simulink model "quad_control_outer_trainingR2015a"  (Simulink 8.5)
settings: Solver=ode45  StartTime=0.0  StopTime=40  FixedStep=0.01  MaxStep=0.1  RelTol=1e-3
InitFcn:
  | % load parameters of the default quadrotor
  | disp('Quadrotor parameters loaded by InitFcn')
  | mdl_quadrotor
  | 
  | % --- Outer loop gains --------
  | %P_X = 3.25;
  | %I_X = 0.45;
  | %D_X = 2;
  | 
  | %P_Y = 2.75;
  | %I_Y = 0.35;
  | %D_Y = 4.75;
  | 
  | %P_Z = 45;
  | %I_Z = 3.5;
  | %D_Z = 25;
  | % --------------------------
  | 
  | rand_ang = pi + (-pi-pi).*rand(1,1);
values from neighbouring files (symbols this model uses):
  D_X = Pitch_controller_coef_escolhidos(3)    [FALA_OUTER_CONTROLLERS.m]    (also in workspace_outer.mat = 3.45)
  D_Y = Roll_controller_coef_escolhidos(3)    [FALA_OUTER_CONTROLLERS.m]    (also in workspace_outer.mat = 3.5)
  D_Z = Yaw_controller_coef_escolhidos(3)    [FALA_OUTER_CONTROLLERS.m]    (also in workspace_outer.mat = 26.7)
  I_X = Pitch_controller_coef_escolhidos(2)    [FALA_OUTER_CONTROLLERS.m]    (also in workspace_outer.mat = 0.16)
  I_Y = Roll_controller_coef_escolhidos(2)    [FALA_OUTER_CONTROLLERS.m]    (also in workspace_outer.mat = 0.04)
  I_Z = Yaw_controller_coef_escolhidos(2)    [FALA_OUTER_CONTROLLERS.m]    (also in workspace_outer.mat = 5.2)
  P_X = Pitch_controller_coef_escolhidos(1)    [FALA_OUTER_CONTROLLERS.m]    (also in workspace_outer.mat = 9.2)
  P_Y = Roll_controller_coef_escolhidos(1)    [FALA_OUTER_CONTROLLERS.m]    (also in workspace_outer.mat = 8.9)
  P_Z = Yaw_controller_coef_escolhidos(1)    [FALA_OUTER_CONTROLLERS.m]    (also in workspace_outer.mat = 53)
  quad =     [workspace_outer.mat]
undefined symbols (not defined in the file or in its folder): sigbuilder_block
libraries: simulink_extras x6, dspsigops x4
settings Model: Creator=corkep  LastModifiedBy=kleber  CovSFcnEnable=off
settings DebuggingCC: SolverPrmCheckMsg=warning  FcnCallInpInsideContextMsg=UseLocalSettings

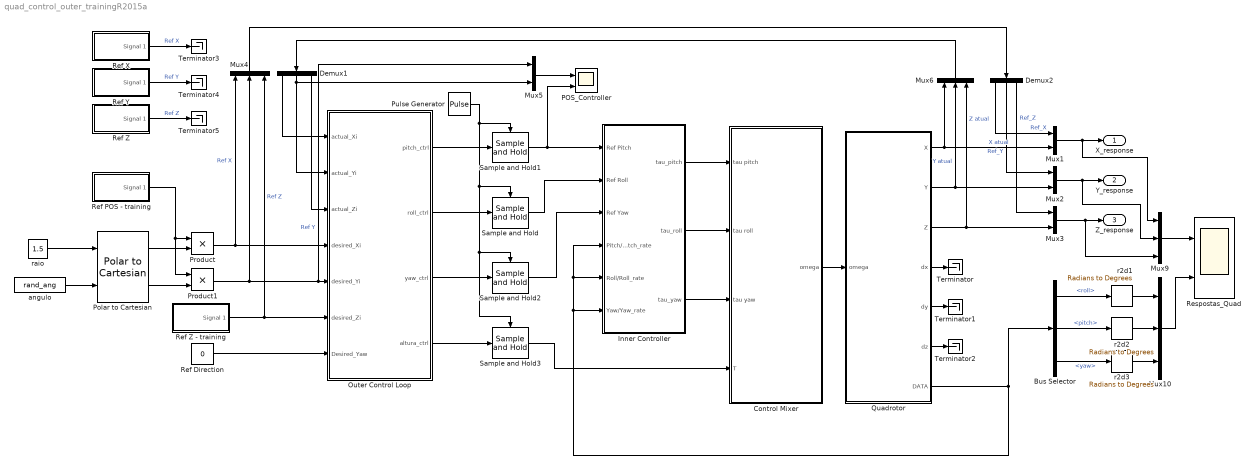
== system quad_control_outer_trainingR2015a ==
  Bus Selector : BusSelector  OutputSignals=roll,pitch,yaw
  Control Mixer : Subsystem  AncestorBlock=roblocks/Dynamics/Control Mixer 4
      mask help: Quadrotor control mixer
      mask Help:
      | Determine rotor speeds based on desired torques and thrust.
      | 
      | <b>Inputs::</b>
      | 
      | tau pitch (1x1)  desired pitching torque [Nm]
      | tau roll (1x1)   desired rolling torque [Nm]
      | tau yaw (1x1)    desired yawing torque [Nm]
      | T (1x1)          desired thrust [N]
      | 
      | <b>Outputs::</b>
      | 
      | w1 (1x1) angular velocity of rotor 1 [rad]
      | w2 (1x1) angular velocity of rotor 2 [rad]
      | w3 (1x1) angular velocity of rotor 3 [rad]
      | w4 (1x1) angular velocity of rotor 4 [rad]
      | 
      | <b>Notes::</b>
      | 
      | - Assumes the rotor labelling convention of RVC Fig 4.16.
      | - The quadrotor is underactuated and has only 4 inputs.
  Demux1 : Demux  Outputs=3
  Demux2 : Demux  Outputs=3
  Inner Controller : Subsystem
  Mux{1..3,5} (4 alike) : Mux  Inputs=2
  Mux10 : Mux  Inputs=3
  Mux4 : Mux  Inputs=3
  Mux6 : Mux  RequirementInfo="{}  %GIDa_c1e701bd_0944_43f7_91ee_3360df493ed1"  Inputs=3
  Mux9 : Mux  Inputs=3
  Outer Control Loop : Subsystem
  POS_Controller : Scope  NumInputPorts=2
      settings: TimeRange=auto  LimitDataPoints=on  MaxDataPoints=5000  SaveToWorkspace=off  SaveName=ScopeData2  YMin=-1.00000~-1.00000  YMax=1.00000~1.00000  SampleTime=-1  DataFormat=Array
  Polar to Cartesian : simulink_extras/Transformations/Polar to Cartesian
  Product : Product
  Product1 : Product
  Pulse Generator : DiscretePulseGenerator  PulseType=Time based  Period=0.1  PulseWidth=10
  Quadrotor : Subsystem  AncestorBlock=roblocks/Dynamics/Quadrotor  mask{quad=quad}
      mask prompts: quad "Quadrotor params"
      mask help: Quadrotor dynamics
      mask Help:
      | Integrate spatial velocity to update pose represented as a homogeneous
      | transformation.
      | 
      | <b>Parameters::</b>
      | 
      | q (struct)  A structure containing quadrotor dynamics
      | 
      | The elements of q are:
      | 
      |  J         Flyer rotational inertia matrix (3x3)
      |  h         Height of rotors above CoG (1x1)
      |  d         Length of flyer arms (1x1)
      |  nb        Number of blades per rotor (1x1)
      |  r         Rotor radius (1x1)
      |  c         Blade chord (1x1)
      |  e         Flapping hinge offset (1x1)
      |  Mb        Rotor blade mass (1x1)
      |  Mc        Estimated hub clamp mass (1x1)
      |  ec        Blade root clamp displacement (1x1)
      |  Ib        Rotor blade rotational inertia (1x1)
      |  Ic        Estimated root clamp inertia (1x1)
      |  mb        Static blade moment (1x1)
      |  Ir        Total rotor inertia (1x1)
      |  Ct        Non-dim. thrust coefficient (1x1)
      |  Cq        Non-dim. torque coefficient (1x1)
      |  sigma     Rotor solidity ratio (1x1)
      |  thetat    Blade tip angle (1x1)
      |  theta0    Blade root angle (1x1)
      |  theta1    Blade twist angle (1x1)
      |  theta75   3/4 blade angle (1x1)
      |  thetai    Blade ideal root approximation (1x1)
      |  a         Lift slope gradient (1x1)
      |  A         Rotor disc area (1x1)
      |  gamma     Lock number (1x1)
      | 
      | 
      | <b>Inputs::</b>
      | 
      | w1 (1x1) angular velocity of rotor 1 [rad]
      | w2 (1x1) angular velocity of rotor 2 [rad]
      | w3 (1x1) angular velocity of rotor 3 [rad]
      | w4 (1x1) angular velocity of rotor 4 [rad]
      | 
      | <b>Outputs::</b>
      | 
      | X (1x12) state vector (x, y, z, thr, thp, thy, xd, yd, zd, thrd, thpd, thyd)
      | 
      | (x,y,z) is the position in the world frame [m]
      | (thr, thp, thy) the roll/pitch/yaw orientation in the world frame [rad]
      | (xd,yd,zd) is the velocity in the body frame [m]
      | (thrd,thpd,thyd) is the roll/pitch/yaw rates in the body frame [rad/s]
      | 
      | <b>Notes::</b>
      | 
      | - See also mdl_quadrotor which defines parameters for the ANU X4 flyer.
  Ref Direction : Constant  Value=0  SampleTime=0
  Ref POS - training : Subsystem  Tag=STV Subsys  LoadFcn=sigbuilder_block('load');  StartFcn=sigbuilder_block('start');  StopFcn=sigbuilder_block('stop');  ClipboardFcn=sigbuilder_block('clipboard');  mask(Sigbuilder block){}
      mask help: Sigbuilder GUI
      mask init:
      | if ~strcmp(get_param(bdroot(gcbh),'SimulationStatus'),'stopped') tuvar = sigbuilder_block('maskInit'); end
      settings: CopyFcn=sigbuilder_block('copy');  DeleteFcn=sigbuilder_block('delete');  ModelCloseFcn=sigbuilder_block('modelClose');  PreSaveFcn=sigbuilder_block('preSave');  PauseFcn=sigbuilder_block('pause')  ContinueFcn=sigbuilder_block('continue')  NameChangeFcn=sigbuilder_block('namechange');  OpenFcn=sigbuilder_block('open',[201 234.75 744 256.5 ]);  CloseFcn=sigbuilder_block('close');
      mask Display: plot(0,0,100,100,[10,10,40,40,10],[80,20,20,80,80],[40,10],[50,50], [40,27,10],[65,72,56],[40,25,25,10],[28,28,43,43]);
  Ref X : Subsystem  Tag=STV Subsys  LoadFcn=sigbuilder_block('load');  StartFcn=sigbuilder_block('start');  StopFcn=sigbuilder_block('stop');  ClipboardFcn=sigbuilder_block('clipboard');  mask(Sigbuilder block){}
      mask help: Sigbuilder GUI
      mask init:
      | if ~strcmp(get_param(bdroot(gcbh),'SimulationStatus'),'stopped') tuvar = sigbuilder_block('maskInit'); end
      settings: CopyFcn=sigbuilder_block('copy');  DeleteFcn=sigbuilder_block('delete');  ModelCloseFcn=sigbuilder_block('modelClose');  PreSaveFcn=sigbuilder_block('preSave');  PauseFcn=sigbuilder_block('pause')  ContinueFcn=sigbuilder_block('continue')  NameChangeFcn=sigbuilder_block('namechange');  OpenFcn=sigbuilder_block('open',[199.5 0 520.5 309.75 ]);  CloseFcn=sigbuilder_block('close');
      mask Display: plot(0,0,100,100,[10,10,40,40,10],[80,20,20,80,80],[40,10],[50,50], [40,27,10],[65,72,56],[40,25,25,10],[28,28,43,43]);
  Ref Y : Subsystem  Tag=STV Subsys  LoadFcn=sigbuilder_block('load');  StartFcn=sigbuilder_block('start');  StopFcn=sigbuilder_block('stop');  ClipboardFcn=sigbuilder_block('clipboard');  mask(Sigbuilder block){}
      mask help: Sigbuilder GUI
      mask init:
      | if ~strcmp(get_param(bdroot(gcbh),'SimulationStatus'),'stopped') tuvar = sigbuilder_block('maskInit'); end
      settings: CopyFcn=sigbuilder_block('copy');  DeleteFcn=sigbuilder_block('delete');  ModelCloseFcn=sigbuilder_block('modelClose');  PreSaveFcn=sigbuilder_block('preSave');  PauseFcn=sigbuilder_block('pause')  ContinueFcn=sigbuilder_block('continue')  NameChangeFcn=sigbuilder_block('namechange');  OpenFcn=sigbuilder_block('open',[268.5 4.5 565.5 444.75 ]);  CloseFcn=sigbuilder_block('close');
      mask Display: plot(0,0,100,100,[10,10,40,40,10],[80,20,20,80,80],[40,10],[50,50], [40,27,10],[65,72,56],[40,25,25,10],[28,28,43,43]);
  Ref Z : Subsystem  Tag=STV Subsys  LoadFcn=sigbuilder_block('load');  StartFcn=sigbuilder_block('start');  StopFcn=sigbuilder_block('stop');  ClipboardFcn=sigbuilder_block('clipboard');  mask(Sigbuilder block){}
      mask help: Sigbuilder GUI
      mask init:
      | if ~strcmp(get_param(bdroot(gcbh),'SimulationStatus'),'stopped') tuvar = sigbuilder_block('maskInit'); end
      settings: CopyFcn=sigbuilder_block('copy');  DeleteFcn=sigbuilder_block('delete');  ModelCloseFcn=sigbuilder_block('modelClose');  PreSaveFcn=sigbuilder_block('preSave');  PauseFcn=sigbuilder_block('pause')  ContinueFcn=sigbuilder_block('continue')  NameChangeFcn=sigbuilder_block('namechange');  OpenFcn=sigbuilder_block('open',[272.25 73.5 542.25 375.75 ]);  CloseFcn=sigbuilder_block('close');
      mask Display: plot(0,0,100,100,[10,10,40,40,10],[80,20,20,80,80],[40,10],[50,50], [40,27,10],[65,72,56],[40,25,25,10],[28,28,43,43]);
  Ref Z - training : Subsystem  Tag=STV Subsys  LoadFcn=sigbuilder_block('load');  StartFcn=sigbuilder_block('start');  StopFcn=sigbuilder_block('stop');  ClipboardFcn=sigbuilder_block('clipboard');  mask(Sigbuilder block){}
      mask help: Sigbuilder GUI
      mask init:
      | if ~strcmp(get_param(bdroot(gcbh),'SimulationStatus'),'stopped') tuvar = sigbuilder_block('maskInit'); end
      settings: CopyFcn=sigbuilder_block('copy');  DeleteFcn=sigbuilder_block('delete');  ModelCloseFcn=sigbuilder_block('modelClose');  PreSaveFcn=sigbuilder_block('preSave');  PauseFcn=sigbuilder_block('pause')  ContinueFcn=sigbuilder_block('continue')  NameChangeFcn=sigbuilder_block('namechange');  OpenFcn=sigbuilder_block('open',[188.25 0 746.25 219.75 ]);  CloseFcn=sigbuilder_block('close');
      mask Display: plot(0,0,100,100,[10,10,40,40,10],[80,20,20,80,80],[40,10],[50,50], [40,27,10],[65,72,56],[40,25,25,10],[28,28,43,43]);
  Respostas_Quad : Scope  NumInputPorts=2
      settings: TimeRange=auto  ShowLegends=on  MaxDataPoints=5000  SaveToWorkspace=off  SaveName=ScopeData  YMin=-0.87795~-1.00000  YMax=1.61055~1.00000  SampleTime=-1  DataFormat=Array
  Sample and Hold{,1..3} (4 alike) : dspsigops/Sample and Hold  trig=Rising edge  initCond=0  latchinput=off
  Terminator{,1..5} (6 alike) : Terminator
  angulo : Constant  Value=rand_ang
  r2d1 : simulink_extras/Transformations/Radians to Degrees
  r2d2 : simulink_extras/Transformations/Radians to Degrees
  r2d3 : simulink_extras/Transformations/Radians to Degrees
  raio : Constant  Value=1.5
  X_response : Outport
  Y_response : Outport  Port=2
  Z_response : Outport  Port=3
  wires:
  Quadrotor/7(DATA) -> Bus Selector/1, Inner Controller/6(Yaw/Yaw_rate), Inner Controller/5(Roll/Roll_rate), Inner Controller/4(Pitch/Pitch_rate)
  Sample and Hold3/1 -> Control Mixer/4(T)
  Control Mixer/1(omega) -> Quadrotor/1(omega)
  Ref Z - training/1(Signal 1) -> Outer Control Loop/6(desired_Zi), Mux4/3  "Ref Z"
  Ref Direction/1 -> Outer Control Loop/7(Desired_Yaw)
  Sample and Hold2/1 -> Inner Controller/3(Ref Yaw)
  Product1/1 -> Mux4/2, Mux5/1, Outer Control Loop/5(desired_Yi)  "Ref Y"
  Mux1/1 -> X_response/1, Mux9/1
  Mux2/1 -> Y_response/1, Mux9/2
  Demux2/1 -> Mux1/1  "Ref_X"
  Demux2/2 -> Mux2/1  "Ref_Y"
  Demux2/3 -> Mux3/1  "Ref_Z"
  Mux4/1 -> Demux2/1
  Outer Control Loop/2(roll_ctrl) -> Sample and Hold/1
  Outer Control Loop/1(pitch_ctrl) -> Sample and Hold1/1
  Outer Control Loop/3(yaw_ctrl) -> Sample and Hold2/1
  Pulse Generator/1 -> Sample and Hold1/Trigger, Sample and Hold/Trigger, Sample and Hold2/Trigger, Sample and Hold3/Trigger
  Outer Control Loop/4(altura_ctrl) -> Sample and Hold3/1
  Mux9/1 -> Respostas_Quad/1
  Mux10/1 -> Respostas_Quad/2
  Bus Selector/2 -> r2d2/1  "<pitch>"
  Bus Selector/1 -> r2d1/1  "<roll>"
  Quadrotor/1(X) -> Mux1/2, Mux6/1  "X atual"
  Quadrotor/3(Z) -> Mux3/2, Mux6/3  "Z atual"
  Bus Selector/3 -> r2d3/1  "<yaw>"
  Quadrotor/2(Y) -> Mux2/2, Mux6/2  "Y atual"
  Sample and Hold/1 -> Inner Controller/2(Ref Roll)
  Sample and Hold1/1 -> POS_Controller/2, Inner Controller/1(Ref Pitch)
  Quadrotor/4(dx) -> Terminator/1
  Quadrotor/5(dy) -> Terminator1/1
  Quadrotor/6(dz) -> Terminator2/1
  Mux5/1 -> POS_Controller/1
  Mux6/1 -> Demux1/1
  Demux1/1 -> Outer Control Loop/1(actual_Xi)
  Demux1/2 -> Outer Control Loop/2(actual_Yi), Mux5/2
  Demux1/3 -> Outer Control Loop/3(actual_Zi)
  Mux3/1 -> Z_response/1, Mux9/3
  Inner Controller/2(tau_roll) -> Control Mixer/2(tau roll)
  Inner Controller/3(tau_yaw) -> Control Mixer/3(tau yaw)
  r2d1/1 -> Mux10/1
  r2d2/1 -> Mux10/2
  r2d3/1 -> Mux10/3
  Inner Controller/1(tau_pitch) -> Control Mixer/1(tau pitch)
  angulo/1 -> Polar to Cartesian/2
  raio/1 -> Polar to Cartesian/1
  Polar to Cartesian/2 -> Product1/2
  Polar to Cartesian/1 -> Product/2
  Ref POS - training/1(Signal 1) -> Product1/1, Product/1
  Ref X/1(Signal 1) -> Terminator3/1  "Ref X"
  Ref Y/1(Signal 1) -> Terminator4/1  "Ref Y"
  Ref Z/1(Signal 1) -> Terminator5/1  "Ref Z"
  Product/1 -> Outer Control Loop/4(desired_Xi), Mux4/1  "Ref X"

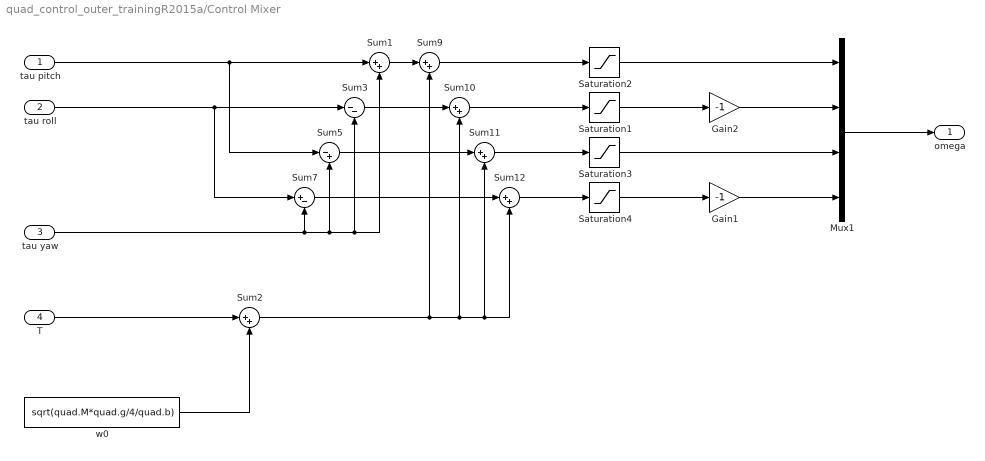
== system quad_control_outer_trainingR2015a/Control Mixer ==
  tau pitch : Inport
  tau roll : Inport  Port=2
  tau yaw : Inport  Port=3
  T : Inport  Port=4
  Gain1 : Gain  Gain=-1
  Gain2 : Gain  Gain=-1
  Mux1 : Mux
  Saturation{1..4} (4 alike) : Saturate  UpperLimit=1000  LowerLimit=700
  Sum{1..2,9..12} (6 alike) : Sum  Inputs=|++  SaturateOnIntegerOverflow=on  InputSameDT=on  OutDataTypeStr=Inherit: Same as first input
  Sum3 : Sum  Inputs=|--  SaturateOnIntegerOverflow=on  InputSameDT=on  OutDataTypeStr=Inherit: Same as first input
  Sum5 : Sum  Inputs=|-+  SaturateOnIntegerOverflow=on  InputSameDT=on  OutDataTypeStr=Inherit: Same as first input
  Sum7 : Sum  Inputs=|+-  SaturateOnIntegerOverflow=on  InputSameDT=on  OutDataTypeStr=Inherit: Same as first input
  w0 : Constant  Value=sqrt(quad.M*quad.g/4/quad.b)  SampleTime=0
  omega : Outport
  wires:
  Mux1/1 -> omega/1
  Gain2/1 -> Mux1/2
  tau yaw/1 -> Sum7/2, Sum5/2, Sum3/2, Sum1/2
  Saturation2/1 -> Mux1/1
  Saturation1/1 -> Gain2/1
  Saturation3/1 -> Mux1/3
  Saturation4/1 -> Gain1/1
  tau pitch/1 -> Sum5/1, Sum1/1
  Sum1/1 -> Sum9/1
  Sum3/1 -> Sum10/1
  Sum5/1 -> Sum11/1
  Sum7/1 -> Sum12/1
  Sum9/1 -> Saturation2/1
  Sum10/1 -> Saturation1/1
  Sum11/1 -> Saturation3/1
  Sum12/1 -> Saturation4/1
  tau roll/1 -> Sum7/1, Sum3/1
  Gain1/1 -> Mux1/4
  Sum2/1 -> Sum9/2, Sum11/2, Sum12/2, Sum10/2
  T/1 -> Sum2/1
  w0/1 -> Sum2/2

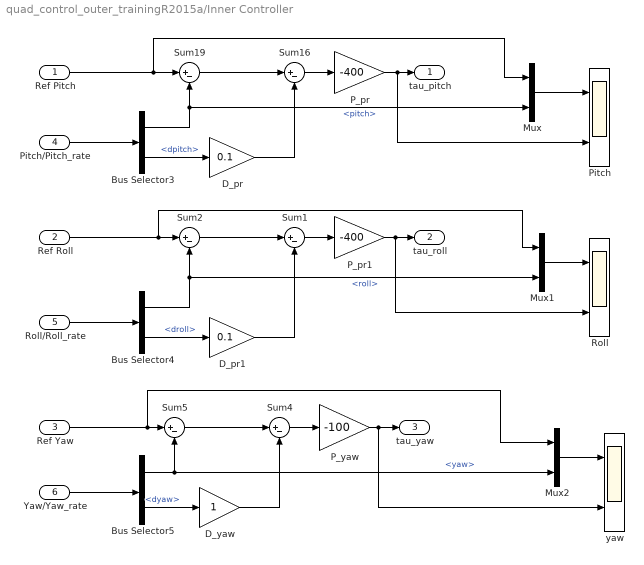
== system quad_control_outer_trainingR2015a/Inner Controller ==
  Ref Pitch : Inport
  Ref Roll : Inport  Port=2
  Ref Yaw : Inport  Port=3
  Pitch/Pitch_rate : Inport  Port=4
  Roll/Roll_rate : Inport  Port=5
  Yaw/Yaw_rate : Inport  Port=6
  Bus Selector3 : BusSelector  OutputSignals=pitch,dpitch
  Bus Selector4 : BusSelector  OutputSignals=roll,droll
  Bus Selector5 : BusSelector  OutputSignals=yaw,dyaw
  D_pr : Gain  Gain=0.1
  D_pr1 : Gain  Gain=0.1
  D_yaw : Gain
  Mux : Mux  Inputs=2
  Mux1 : Mux  Inputs=2
  Mux2 : Mux  Inputs=2
  P_pr : Gain  Gain=-400
  P_pr1 : Gain  Gain=-400
  P_yaw : Gain  Gain=-100
  Pitch : Scope  NumInputPorts=2
      settings: TimeRange=auto  LimitDataPoints=on  MaxDataPoints=5000  SaveToWorkspace=off  SaveName=ScopeData  YMin=-0.0125~-0.7  YMax=0.0175~0.6  SampleTime=-1  DataFormat=Array
  Roll : Scope  NumInputPorts=2
      settings: TimeRange=auto  LimitDataPoints=on  MaxDataPoints=5000  SaveToWorkspace=off  SaveName=ScopeData  YMin=-0.01734~-5.23317  YMax=0.01577~5.91532  SampleTime=-1  DataFormat=Array
  Sum{1..2,4..5,16,19} (6 alike) : Sum  Inputs=|+-
  yaw : Scope  NumInputPorts=2
      settings: TimeRange=auto  LimitDataPoints=on  MaxDataPoints=5000  SaveToWorkspace=off  YMin=-0.03214~-3.77778  YMax=0.02077~2.90017  SampleTime=-1  DataFormat=Array
  tau_pitch : Outport
  tau_roll : Outport  Port=2
  tau_yaw : Outport  Port=3
  wires:
  Sum19/1 -> Sum16/1
  Sum16/1 -> P_pr/1
  P_pr/1 -> Pitch/2, tau_pitch/1
  D_pr/1 -> Sum16/2
  Bus Selector3/2 -> D_pr/1  "<dpitch>"
  Bus Selector3/1 -> Sum19/2, Mux/2  "<pitch>"
  Sum2/1 -> Sum1/1
  Sum1/1 -> P_pr1/1
  P_pr1/1 -> Roll/2, tau_roll/1
  D_pr1/1 -> Sum1/2
  Bus Selector4/2 -> D_pr1/1  "<droll>"
  Ref Pitch/1 -> Mux/1, Sum19/1
  Pitch/Pitch_rate/1 -> Bus Selector3/1
  Roll/Roll_rate/1 -> Bus Selector4/1
  Bus Selector4/1 -> Mux1/2, Sum2/2  "<roll>"
  Ref Roll/1 -> Mux1/1, Sum2/1
  Bus Selector5/1 -> Sum5/2, Mux2/2  "<yaw>"
  Sum4/1 -> P_yaw/1
  Bus Selector5/2 -> D_yaw/1  "<dyaw>"
  D_yaw/1 -> Sum4/2
  Sum5/1 -> Sum4/1
  P_yaw/1 -> yaw/2, tau_yaw/1
  Yaw/Yaw_rate/1 -> Bus Selector5/1
  Ref Yaw/1 -> Mux2/1, Sum5/1
  Mux/1 -> Pitch/1
  Mux1/1 -> Roll/1
  Mux2/1 -> yaw/1

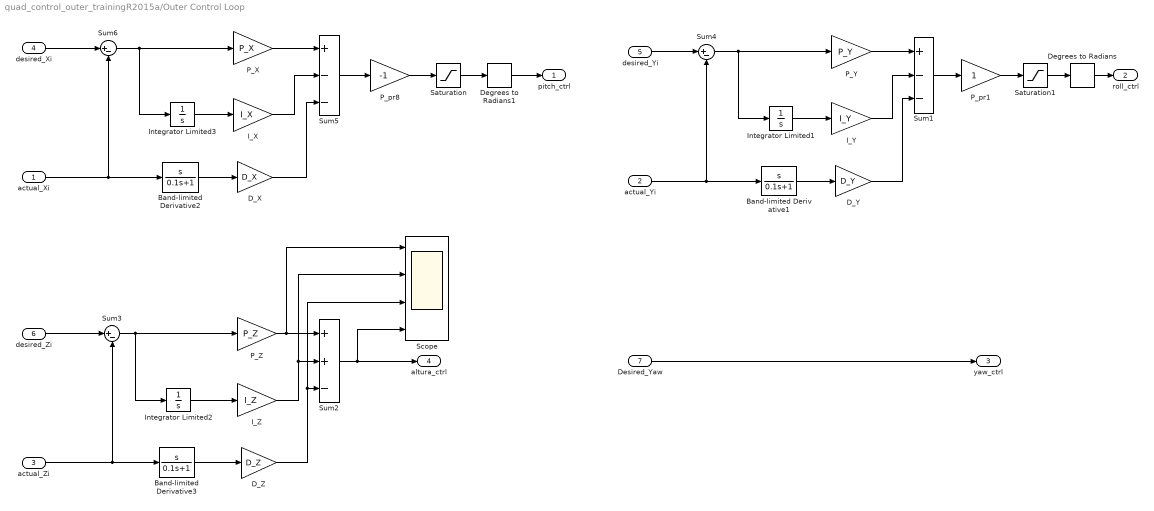
== system quad_control_outer_trainingR2015a/Outer Control Loop ==
  actual_Xi : Inport
  actual_Yi : Inport  Port=2
  actual_Zi : Inport  Port=3
  desired_Xi : Inport  Port=4
  desired_Yi : Inport  Port=5
  desired_Zi : Inport  Port=6
  Desired_Yaw : Inport  Port=7
  Band-limited Deriv ative1 : TransferFcn  Numerator=[1 0]  Denominator=[0.1 1]
  Band-limited Derivative2 : TransferFcn  Numerator=[1 0]  Denominator=[0.1 1]
  Band-limited Derivative3 : TransferFcn  Numerator=[1 0]  Denominator=[0.1 1]
  D_X : Gain  Gain=D_X
  D_Y : Gain  Gain=D_Y
  D_Z : Gain  Gain=D_Z
  Degrees to Radians : simulink_extras/Transformations/Degrees to Radians
  Degrees to Radians1 : simulink_extras/Transformations/Degrees to Radians
  I_X : Gain  Gain=I_X
  I_Y : Gain  Gain=I_Y
  I_Z : Gain  Gain=I_Z
  Integrator Limited1 : Integrator  LimitOutput=on  UpperSaturationLimit=0.5  LowerSaturationLimit=-0.5
  Integrator Limited2 : Integrator  LimitOutput=on  UpperSaturationLimit=10  LowerSaturationLimit=0
  Integrator Limited3 : Integrator  LimitOutput=on  UpperSaturationLimit=0.5  LowerSaturationLimit=-0.5
  P_X : Gain  Gain=P_X
  P_Y : Gain  Gain=P_Y
  P_Z : Gain  Gain=P_Z
  P_pr1 : Gain
  P_pr8 : Gain  Gain=-1
  Saturation : Saturate  UpperLimit=2  LowerLimit=-2
  Saturation1 : Saturate  UpperLimit=2  LowerLimit=-2
  Scope : Scope  NumInputPorts=4
      settings: TimeRange=auto  MaxDataPoints=5000  SaveToWorkspace=off  YMin=3.53924~-5.84467~-1.00000~-2.30544  YMax=26.72734~52.60207~1.00000~79.32941  SampleTime=-1
  Sum1 : Sum  Inputs=+--
  Sum2 : Sum  Inputs=++-
  Sum3 : Sum  Inputs=|+-
  Sum4 : Sum  Inputs=|+-
  Sum5 : Sum  Inputs=+--
  Sum6 : Sum  Inputs=|+-
  pitch_ctrl : Outport
  roll_ctrl : Outport  Port=2
  yaw_ctrl : Outport  Port=3
  altura_ctrl : Outport  Port=4
  wires:
  Sum3/1 -> Integrator Limited2/1, P_Z/1
  Integrator Limited2/1 -> I_Z/1
  P_Z/1 -> Sum2/1, Scope/1
  D_Z/1 -> Scope/3, Sum2/3
  actual_Zi/1 -> Sum3/2, Band-limited Derivative3/1
  Band-limited Derivative3/1 -> D_Z/1
  desired_Zi/1 -> Sum3/1
  Desired_Yaw/1 -> yaw_ctrl/1
  Sum6/1 -> Integrator Limited3/1, P_X/1
  Integrator Limited3/1 -> I_X/1
  P_X/1 -> Sum5/1
  D_X/1 -> Sum5/3
  actual_Xi/1 -> Band-limited Derivative2/1, Sum6/2
  Band-limited Derivative2/1 -> D_X/1
  desired_Xi/1 -> Sum6/1
  I_X/1 -> Sum5/2
  Sum4/1 -> Integrator Limited1/1, P_Y/1
  Integrator Limited1/1 -> I_Y/1
  P_Y/1 -> Sum1/1
  D_Y/1 -> Sum1/3
  actual_Yi/1 -> Sum4/2, Band-limited Deriv ative1/1
  Band-limited Deriv ative1/1 -> D_Y/1
  desired_Yi/1 -> Sum4/1
  I_Y/1 -> Sum1/2
  Degrees to Radians/1 -> roll_ctrl/1
  Degrees to Radians1/1 -> pitch_ctrl/1
  Sum1/1 -> P_pr1/1
  I_Z/1 -> Sum2/2, Scope/2
  Sum5/1 -> P_pr8/1
  Sum2/1 -> Scope/4, altura_ctrl/1
  P_pr8/1 -> Saturation/1
  Saturation/1 -> Degrees to Radians1/1
  P_pr1/1 -> Saturation1/1
  Saturation1/1 -> Degrees to Radians/1

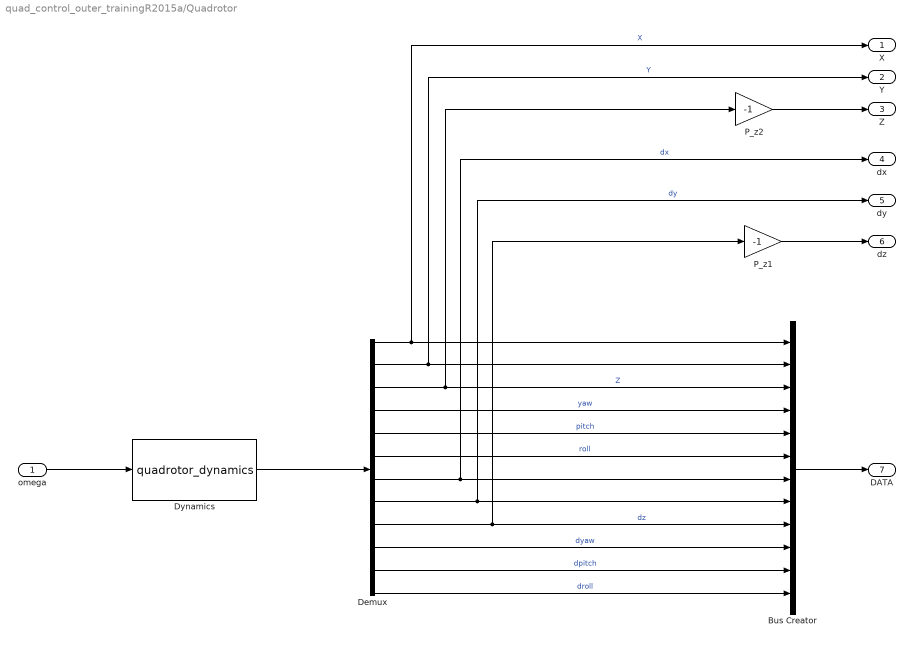
== system quad_control_outer_trainingR2015a/Quadrotor ==
  omega : Inport
  Bus Creator : BusCreator  Inputs='X','Y','Z','yaw','pitch','roll','dx','dy','dz','dyaw','dpitch','droll'
  Demux : Demux  Outputs=12
  Dynamics : S-Function  FunctionName=quadrotor_dynamics  Parameters=quad  SFunctionDeploymentMode=off  EnableBusSupport=off
  P_z1 : Gain  Gain=-1
  P_z2 : Gain  Gain=-1
  X : Outport
  Y : Outport  Port=2
  Z : Outport  Port=3
  dx : Outport  Port=4
  dy : Outport  Port=5
  dz : Outport  Port=6
  DATA : Outport  Port=7
  wires:
  Demux/1 -> X/1, Bus Creator/1  "X"
  Demux/3 -> Bus Creator/3, P_z2/1  "Z"
  Demux/4 -> Bus Creator/4  "yaw"
  Demux/5 -> Bus Creator/5  "pitch"
  omega/1 -> Dynamics/1
  Demux/7 -> dx/1, Bus Creator/7  "dx"
  Demux/9 -> P_z1/1, Bus Creator/9  "dz"
  Demux/2 -> Y/1, Bus Creator/2  "Y"
  Demux/6 -> Bus Creator/6  "roll"
  Demux/8 -> dy/1, Bus Creator/8  "dy"
  Bus Creator/1 -> DATA/1
  Dynamics/1 -> Demux/1
  Demux/10 -> Bus Creator/10  "dyaw"
  Demux/11 -> Bus Creator/11  "dpitch"
  Demux/12 -> Bus Creator/12  "droll"
  P_z2/1 -> Z/1
  P_z1/1 -> dz/1

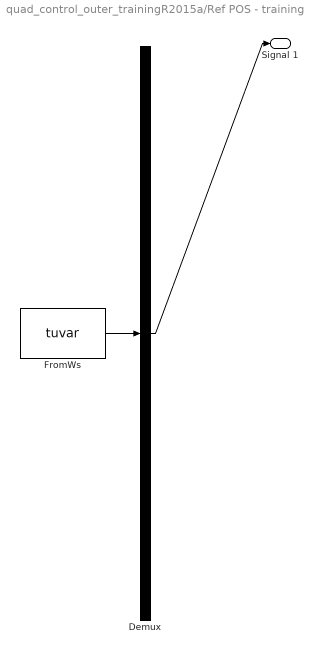
== system quad_control_outer_trainingR2015a/Ref POS - training ==
  Demux : Demux  Tag=STV Demux  Outputs=1
  FromWs : FromWorkspace  Tag=STV FromWs  VariableName=tuvar  SampleTime=0  SigBuilderData=DataTag0  VnvData=DataTag1
      SigBuilderData=|
      | common.afterFinalStr = 'Extrapolate'
      | common.sampleTime = 0
      | dataSet.timeRange = [0 40]
      | dataSet.name = 'Group 1'
      | sbobj.Name = 'Signal Builder'
      | sbobj.Groups.Name = 'Group 1'
      | sbobj.Groups.Signals.Name = 'Signal 1'
      | sbobj.Groups.Signals.XData = [0 5 15 15 40]
      | sbobj.Groups.Signals.YData = [0 0 1 1 1]
      | sbobj.Groups.TimeRange = [0 40]
  Signal 1 : Outport  Tag=STV Outport
  wires:
  Demux/1 -> Signal 1/1
  FromWs/1 -> Demux/1

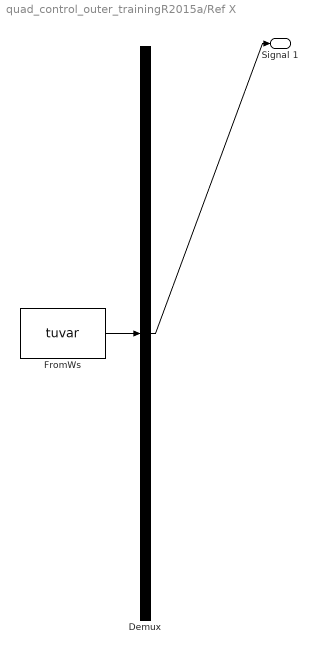
== system quad_control_outer_trainingR2015a/Ref X ==
  Demux : Demux  Tag=STV Demux  Outputs=1
  FromWs : FromWorkspace  Tag=STV FromWs  VariableName=tuvar  SampleTime=0  SigBuilderData=DataTag2  VnvData=DataTag3
      SigBuilderData=|
      | common.afterFinalStr = 'Extrapolate'
      | common.sampleTime = 0
      | dataSet.timeRange = [0 30]
      | dataSet.name = 'Group 1'
      | sbobj.Name = 'Signal Builder'
      | sbobj.Groups.Name = 'Group 1'
      | sbobj.Groups.Signals.Name = 'Signal 1'
      | sbobj.Groups.Signals.XData = [0 10 15 30]
      | sbobj.Groups.Signals.YData = [0 0 1 1]
      | sbobj.Groups.TimeRange = [0 30]
  Signal 1 : Outport  Tag=STV Outport
  wires:
  FromWs/1 -> Demux/1
  Demux/1 -> Signal 1/1

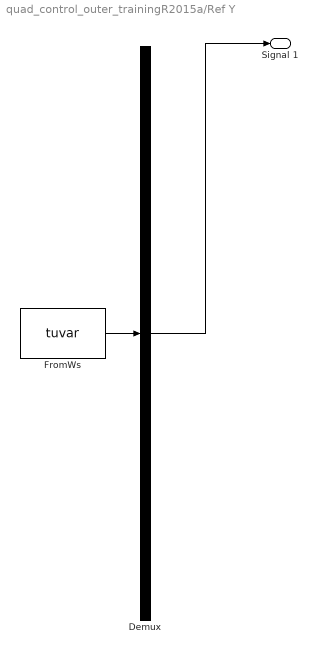
== system quad_control_outer_trainingR2015a/Ref Y ==
  Demux : Demux  Tag=STV Demux  Outputs=1
  FromWs : FromWorkspace  Tag=STV FromWs  VariableName=tuvar  SampleTime=0  SigBuilderData=DataTag4  VnvData=DataTag5
      SigBuilderData=|
      | common.afterFinalStr = 'Extrapolate'
      | common.sampleTime = 0
      | dataSet.timeRange = [0 30]
      | dataSet.name = 'Group 1'
      | sbobj.Name = 'Signal Builder'
      | sbobj.Groups.Name = 'Group 1'
      | sbobj.Groups.Signals.Name = 'Signal 1'
      | sbobj.Groups.Signals.XData = [0 5 10 30]
      | sbobj.Groups.Signals.YData = [0 0 1.5 1.5]
      | sbobj.Groups.TimeRange = [0 30]
  Signal 1 : Outport  Tag=STV Outport
  wires:
  Demux/1 -> Signal 1/1
  FromWs/1 -> Demux/1

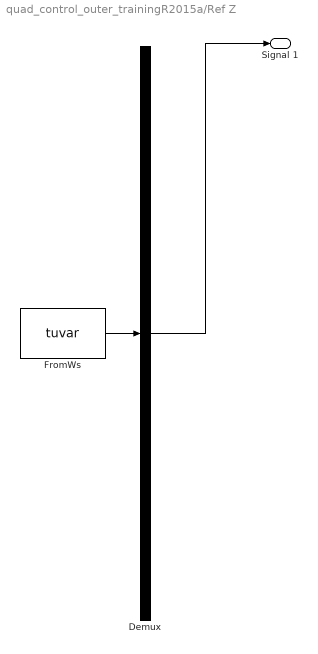
== system quad_control_outer_trainingR2015a/Ref Z ==
  Demux : Demux  Tag=STV Demux  Outputs=1
  FromWs : FromWorkspace  Tag=STV FromWs  VariableName=tuvar  SampleTime=0  SigBuilderData=DataTag6  VnvData=DataTag7
      SigBuilderData=|
      | common.afterFinalStr = 'Extrapolate'
      | common.sampleTime = 0
      | dataSet.timeRange = [0 50]
      | dataSet.name = 'Group 1'
      | sbobj.Name = 'Signal Builder'
      | sbobj.Groups.Name = 'Group 1'
      | sbobj.Groups.Signals.Name = 'Signal 1'
      | sbobj.Groups.Signals.XData = [0 2.5 20 40 50]
      | sbobj.Groups.Signals.YData = [0 2 2 2 2]
      | sbobj.Groups.TimeRange = [0 50]
  Signal 1 : Outport  Tag=STV Outport
  wires:
  Demux/1 -> Signal 1/1
  FromWs/1 -> Demux/1

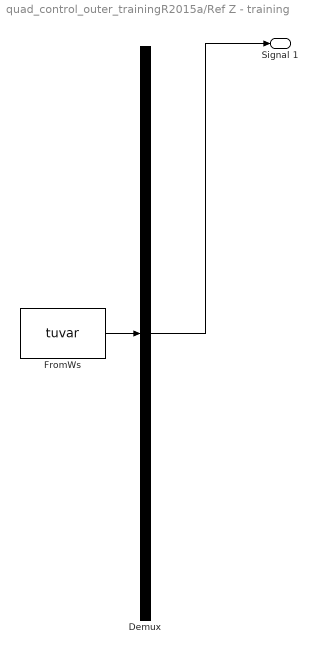
== system quad_control_outer_trainingR2015a/Ref Z - training ==
  Demux : Demux  Tag=STV Demux  Outputs=1
  FromWs : FromWorkspace  Tag=STV FromWs  VariableName=tuvar  SampleTime=0  SigBuilderData=DataTag8  VnvData=DataTag9
      SigBuilderData=|
      | common.afterFinalStr = 'Extrapolate'
      | common.sampleTime = 0
      | dataSet.timeRange = [0 40]
      | dataSet.name = 'Group 1'
      | sbobj.Name = 'Signal Builder'
      | sbobj.Groups.Name = 'Group 1'
      | sbobj.Groups.Signals.Name = 'Signal 1'
      | sbobj.Groups.Signals.XData = [0 5 20 25 30 35 40]
      | sbobj.Groups.Signals.YData = [0.12 0.5 0.5 0.15 0.15 0.5 0.5]
      | sbobj.Groups.TimeRange = [0 40]
  Signal 1 : Outport  Tag=STV Outport
  wires:
  FromWs/1 -> Demux/1
  Demux/1 -> Signal 1/1
